simulink model "primjerC"  (R2023a)
settings: Solver=VariableStepAuto  StartTime=0.0  StopTime=20  RelTol=1e-3
InitFcn:
  | clear mex
values from neighbouring files (symbols this model uses):
  Gpid_D_FI_1 = tf(num_fi, den_fi, Ts1)    [controller.m]
  Gpid_D_FI_2 = tf(num2_fi, den2_fi, Ts2)    [controller.m]
  Gpid_D_S1_FI_3 = tf(num3_fi, den3_fi, Ts1)    [controller.m]
  Gpid_D_S1_FI_5 = tf(num5_fi, den5_fi, Ts2)    [controller.m]
  Gpid_D_S2_FI_4 = tf(num4_fi, den4_fi, Ts1)    [controller.m]
  Gpid_D_S2_FI_6 = tf(num6_fi, den6_fi, Ts2)    [controller.m]
  Ts1 = 0.03    [controller.m]
  Ts2 = 0.005    [controller.m]
undefined symbols (not defined in the file or in its folder): den1, den2, den_pid, num1, num2, num_pid
settings Model: Creator=Sandor  LastModifiedBy=Enio
settings DebuggingCC: UnconnectedInputMsg=warning  UnconnectedOutputMsg=warning  UnconnectedLineMsg=warning
settings ModelReferenceCC: EnableRefExpFcnMdlSchedulingChecks=on
settings SFSimCC: SimCustomHeaderCode="#include \"controller.h\""  SimUserSources=controller.c
settings RTWCC: DLArmComputeVersion=19.05

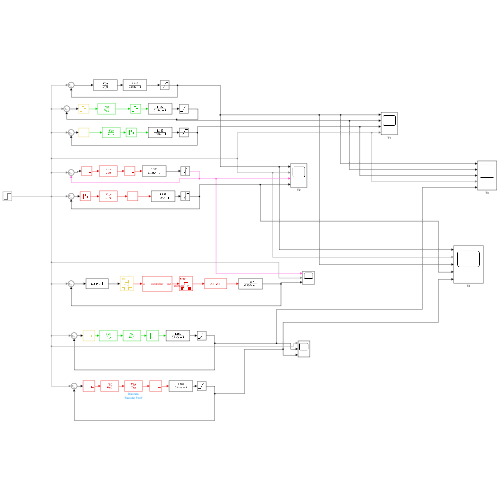
[thumbnail: Simulink's stored preview of the top-level diagram]
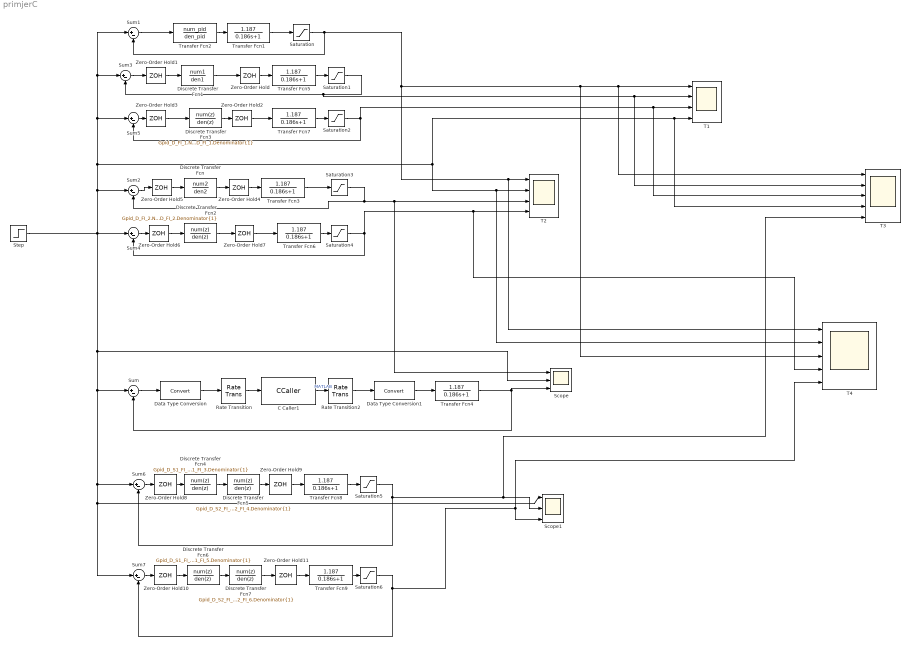
== system primjerC ==
  C Caller1 : CCaller  FunctionName=controller  PortSpecificationStruct="%)30     .    N ,   8    (     @         %    \"     (    !     0         %  0 \"0    $    _    07)G3F%M90  4&]R=$YA;64 4V-O<&4     26YD97@     5'EP90      4VEZ90      27-';&]B86P   X    P    !@    @    $          4    (     0    ,    !         !   P!O=70 #@   #     &    \"     0         !0    @    !     P    $         $  # &]U=  .    .     8    (    !          %    \"     $    &     0         0    !@   $]U='!U=   #@   #@    &    \"     8         !0    @    !     0    $         \"0    @               X    X    !@    @    $          4    (     0    8    !         !     &    <VEN9VQE   .    ,     8    (    !          %    \"     $    !     0         0  $ ,0    X    P    !@    @    ) @        4    (     0    $    !          (  0      #@   #     &    \"     0         !0    @    !     0    $         $  ! '4    .    ,     8    (    !          %    \"     $    !     0         0  $ =0    X    X    !@    @    $          4    (     0    4    !         !     %    26YP=70    .    .     8    (    !@         %    \"     $    !     0         )    \"               #@   #@    &    \"     0         !0    @    !    !@    $         $     8   !S:6YG;&4   X    P    !@    @    $          4    (     0    $    !         !   0 Q    #@   #     &    \"     D\"        !0    @    !     0    $          @ !"
  Data Type Conversion : DataTypeConversion  SaturateOnIntegerOverflow=off  RndMeth=Floor
  Data Type Conversion1 : DataTypeConversion  SaturateOnIntegerOverflow=off  RndMeth=Floor
  Discrete Transfer Fcn : DiscreteTransferFcn  Numerator=num2  Denominator=den2  SampleTime=Ts2
  Discrete Transfer Fcn1 : DiscreteTransferFcn  Numerator=num1  Denominator=den1
  Discrete Transfer Fcn2 : DiscreteTransferFcn  Numerator=Gpid_D_FI_2.Numerator{1}  Denominator=Gpid_D_FI_2.Denominator{1}  SampleTime=Ts2
  Discrete Transfer Fcn3 : DiscreteTransferFcn  Numerator=Gpid_D_FI_1.Numerator{1}  Denominator=Gpid_D_FI_1.Denominator{1}
  Discrete Transfer Fcn4 : DiscreteTransferFcn  Numerator=Gpid_D_S1_FI_3.Numerator{1}  Denominator=Gpid_D_S1_FI_3.Denominator{1}
  Discrete Transfer Fcn5 : DiscreteTransferFcn  Numerator=Gpid_D_S2_FI_4.Numerator{1}  Denominator=Gpid_D_S2_FI_4.Denominator{1}
  Discrete Transfer Fcn6 : DiscreteTransferFcn  Numerator=Gpid_D_S1_FI_5.Numerator{1}  Denominator=Gpid_D_S1_FI_5.Denominator{1}
  Discrete Transfer Fcn7 : DiscreteTransferFcn  Numerator=Gpid_D_S2_FI_6.Numerator{1}  Denominator=Gpid_D_S2_FI_6.Denominator{1}
  Rate Transition : RateTransition  OutPortSampleTime=Ts2
  Rate Transition2 : RateTransition  OutPortSampleTime=Ts2
  Saturation{,1..6} (7 alike) : Saturate  UpperLimit=10  LowerLimit=-6
  Scope : Scope  NumInputPorts=3
  Scope1 : Scope  NumInputPorts=3
  Step : Step  After=6  SampleTime=0
  Sum{,1..7} (8 alike) : Sum  Inputs=|+-
  T1 : Scope  NumInputPorts=4
  T2 : Scope  NumInputPorts=4
  T3 : Scope  NumInputPorts=5
  T4 : Scope  NumInputPorts=5
  Transfer Fcn{1,3..9} (8 alike) : TransferFcn  Numerator=[1.187]  Denominator=[0.186 1]
  Transfer Fcn2 : TransferFcn  Numerator=num_pid  Denominator=den_pid
  Zero-Order Hold{,1..3,8..9} (6 alike) : ZeroOrderHold  SampleTime=Ts1
  Zero-Order Hold{4..7,10..11} (6 alike) : ZeroOrderHold  SampleTime=Ts2
  wires:
  Rate Transition/1 -> C Caller1/1
  Data Type Conversion/1 -> Rate Transition/1
  Sum/1 -> Data Type Conversion/1
  Sum1/1 -> Transfer Fcn2/1
  Transfer Fcn2/1 -> Transfer Fcn1/1
  Transfer Fcn1/1 -> Saturation/1
  Saturation/1 -> T4/1, T2/1, T4/3, T3/1, T1/1, Sum1/2
  Transfer Fcn5/1 -> Saturation1/1
  Saturation1/1 -> T3/2, T1/2, Sum3/2
  Transfer Fcn7/1 -> Saturation2/1
  Saturation2/1 -> T3/3, T1/3, Sum5/2
  Transfer Fcn3/1 -> Saturation3/1
  Transfer Fcn6/1 -> Saturation4/1
  Saturation4/1 -> T4/4, T2/4, Sum4/2
  Saturation5/1 -> Sum6/2, T3/5, Scope1/2
  Transfer Fcn8/1 -> Saturation5/1
  Discrete Transfer Fcn4/1 -> Discrete Transfer Fcn5/1
  Saturation6/1 -> T4/5, Scope1/3, Sum7/2
  Discrete Transfer Fcn6/1 -> Discrete Transfer Fcn7/1
  Transfer Fcn9/1 -> Saturation6/1
  Step/1 -> Scope1/1, Sum7/1, Sum6/1, Sum/1, Scope/2, T4/2, T2/2, T3/4, T1/4, Sum5/1, Sum3/1, Sum1/1, Sum2/1, Sum4/1
  Zero-Order Hold/1 -> Transfer Fcn5/1
  Discrete Transfer Fcn1/1 -> Zero-Order Hold/1
  Zero-Order Hold1/1 -> Discrete Transfer Fcn1/1
  Sum3/1 -> Zero-Order Hold1/1
  Zero-Order Hold2/1 -> Transfer Fcn7/1
  Discrete Transfer Fcn3/1 -> Zero-Order Hold2/1
  Sum5/1 -> Zero-Order Hold3/1
  Zero-Order Hold3/1 -> Discrete Transfer Fcn3/1
  Discrete Transfer Fcn/1 -> Zero-Order Hold4/1
  Zero-Order Hold4/1 -> Transfer Fcn3/1
  Zero-Order Hold5/1 -> Discrete Transfer Fcn/1
  Sum2/1 -> Zero-Order Hold5/1
  Sum4/1 -> Zero-Order Hold6/1
  Zero-Order Hold6/1 -> Discrete Transfer Fcn2/1
  Discrete Transfer Fcn2/1 -> Zero-Order Hold7/1
  Zero-Order Hold7/1 -> Transfer Fcn6/1
  Transfer Fcn4/1 -> Scope/3, Sum/2
  Zero-Order Hold8/1 -> Discrete Transfer Fcn4/1
  Sum6/1 -> Zero-Order Hold8/1
  Zero-Order Hold9/1 -> Transfer Fcn8/1
  Discrete Transfer Fcn5/1 -> Zero-Order Hold9/1
  Sum7/1 -> Zero-Order Hold10/1
  Zero-Order Hold10/1 -> Discrete Transfer Fcn6/1
  Zero-Order Hold11/1 -> Transfer Fcn9/1
  Discrete Transfer Fcn7/1 -> Zero-Order Hold11/1
  Data Type Conversion1/1 -> Transfer Fcn4/1
  Rate Transition2/1 -> Data Type Conversion1/1
  C Caller1/1 -> Rate Transition2/1  "MATLAB"
  Saturation3/1 -> Scope/1, T2/3, Sum2/2
